simulink model "ANC_simulink_2"  (R2023b)
settings: Solver=VariableStepAuto  StartTime=0.0  StopTime=1  RelTol=1e-3
values from neighbouring files (symbols this model uses):
  A = 10    [parameter.mat]
  c = 343    [parameter.mat]
  f = 10    [parameter.mat]
  Lp = 1    [parameter.mat]
  Ls = 0.1    [parameter.mat]
  Ts = 0.001    [parameter.mat]
settings Model: Creator=nurbi  LastModifiedBy=nurbi

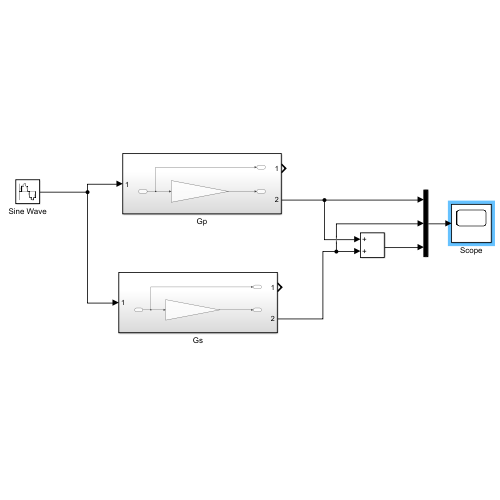
[thumbnail: Simulink's stored preview of the top-level diagram]
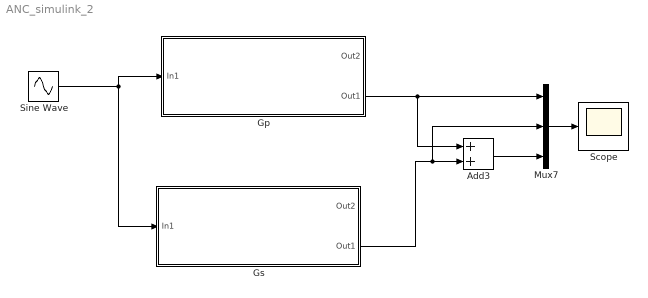
== system ANC_simulink_2 ==
  Add3 : Sum
  Gp : Subsystem
  Gs : Subsystem
  Mux7 : Mux  Inputs=3
  Scope : Scope
  Sine Wave : Sin  Amplitude=A  Frequency=2*pi*f  SampleTime=Ts
  wires:
  Sine Wave/1 -> Gs/1(In1), Gp/1(In1)
  Gp/2(Out1) -> Add3/1, Mux7/1
  Gs/2(Out1) -> Mux7/2, Add3/2
  Mux7/1 -> Scope/1
  Add3/1 -> Mux7/3

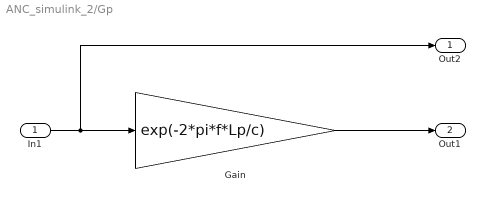
== system ANC_simulink_2/Gp ==
  In1 : Inport
  Gain : Gain  Gain=exp(-2*pi*f*Lp/c)
  Out2 : Outport
  Out1 : Outport  Port=2
  wires:
  In1/1 -> Out2/1, Gain/1
  Gain/1 -> Out1/1

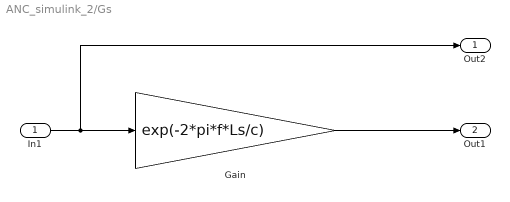
== system ANC_simulink_2/Gs ==
  In1 : Inport
  Gain : Gain  Gain=exp(-2*pi*f*Ls/c)
  Out2 : Outport
  Out1 : Outport  Port=2
  wires:
  In1/1 -> Out2/1, Gain/1
  Gain/1 -> Out1/1
